simulink model "que5_2"  (R2023a)
settings: Solver=VariableStepAuto  StartTime=0.0  StopTime=150  RelTol=1e-3
values from neighbouring files (symbols this model uses):
  A = [0 1 0 0 ... (first row only)    [que5_1.m]    (also in que5_1_1.m; que5_4.m; que6_1.m = [0 1 0; que6_2_sim_input.m = [0 1 0;0 0 1;0 0 -0.5])
  B = [0 ... (first row only)    [que5_1.m]    (also in que5_1_1.m; que5_4.m; que6_1.m = [0 0 0.5]'; que6_2_sim_input.m = [0;0;0.5])
  C = [1,0, 0, 0 ... (first row only)    [que5_1.m]    (also in que5_1_1.m; que5_4.m = [1, 0, 0, 0]; que6_1.m = [1 0 0; que6_2_sim_input.m = [1 0 0)
  g = 9.8    [que5_1.m]    (also in que5_1_1.m; que5_4.m)
  I = 1/3*m*l^2    (= 0.00833333333333)    [que5_1.m]    (also in que5_1_1.m; que5_4.m)
  l = 0.5    [que5_1.m]    (also in que5_1_1.m; que5_4.m)
  m = 0.1    [que5_1.m]    (also in que5_1_1.m; que5_4.m)
  M = 2    [que5_1.m]    (also in que5_1_1.m; que5_4.m)
settings Model: Creator=Hasee  LastModifiedBy=Administrator

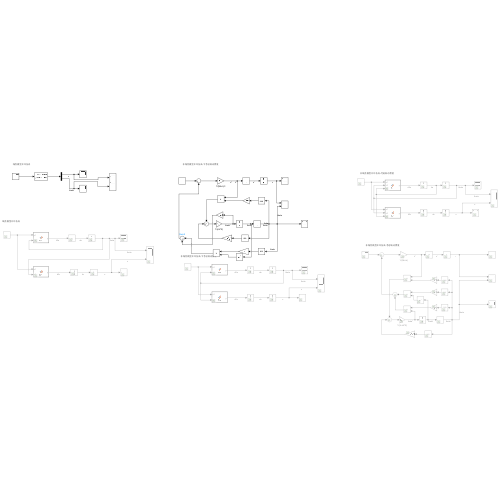
[thumbnail: Simulink's stored preview of the top-level diagram]
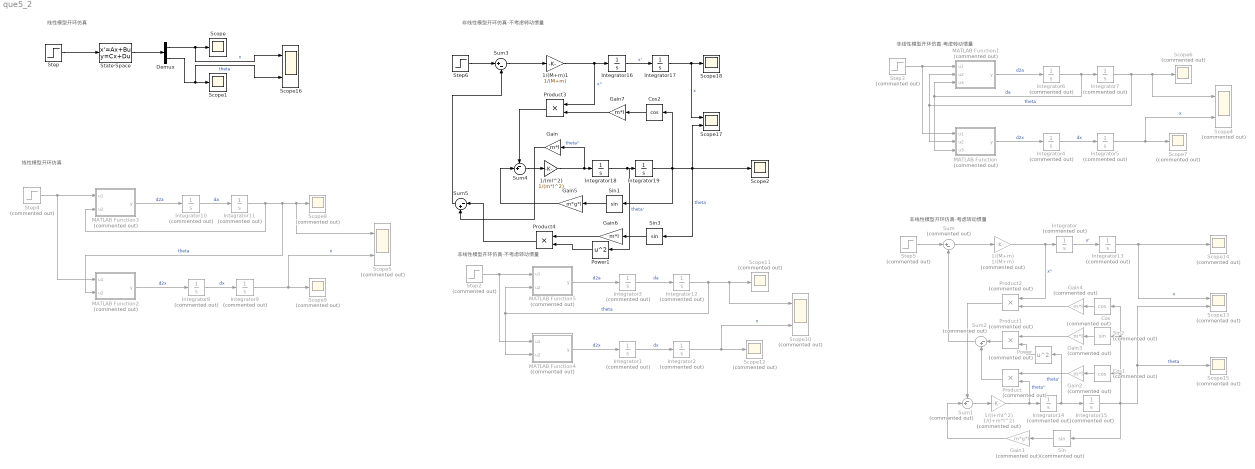
== system que5_2 ==
  note: 线性模型开环仿真
  note: 线性模型开环仿真
  note: 非线性模型开环仿真-不考虑转动惯量
  note: 非线性模型开环仿真-不考虑转动惯量
  note: 非线性模型开环仿真-考虑转动惯量
  note: 非线性模型开环仿真-考虑转动惯量
  1/(I+ml^2) : Gain  Commented=on  Gain=1/(I+m*l^2)
  1/(M+m) : Gain  Commented=on  Gain=1/(M+m)
  1/(M+m)1 : Gain  Gain=1/(M+m)
  1/(ml^2) : Gain  Gain=1/(m*l^2)
  Cos : Trigonometry  Commented=on  Operator=cos
  Cos1 : Trigonometry  Commented=on  Operator=cos
  Cos2 : Trigonometry  Operator=cos
  Demux : Demux  Outputs=2
  Gain : Gain  Gain=m*l
  Gain1 : Gain  Commented=on  Gain=m*g*l
  Gain2 : Gain  Commented=on  Gain=m*l
  Gain3 : Gain  Commented=on  Gain=m*l
  Gain4 : Gain  Commented=on  Gain=m*l
  Gain5 : Gain  Gain=m*g*l
  Gain6 : Gain  Gain=m*l
  Gain7 : Gain  Gain=m*l
  Integrator{,1..15} (16 alike) : Integrator  Commented=on
  Integrator{16..19} (4 alike) : Integrator
  MATLAB Function : MATLAB Function  Commented=on  TreatAsAtomicUnit=on
  MATLAB Function1 : MATLAB Function  Commented=on  TreatAsAtomicUnit=on
  MATLAB Function2 : MATLAB Function  Commented=on  TreatAsAtomicUnit=on
  MATLAB Function3 : MATLAB Function  Commented=on  TreatAsAtomicUnit=on
  MATLAB Function4 : MATLAB Function  Commented=on  TreatAsAtomicUnit=on
  MATLAB Function5 : MATLAB Function  Commented=on  TreatAsAtomicUnit=on
  Power : Math  Commented=on  Operator=square
  Power1 : Math  Operator=square
  Product : Product  Commented=on
  Product1 : Product  Commented=on
  Product2 : Product  Commented=on
  Product3 : Product
  Product4 : Product
  Scope{,1..2,18} (4 alike) : Scope
  Scope{4..5,10,13} (4 alike) : Scope  Commented=on  NumInputPorts=2
  Scope{6..9,11..12,14..15} (8 alike) : Scope  Commented=on
  Scope16 : Scope  NumInputPorts=2
  Scope17 : Scope  NumInputPorts=2
  Sin : Trigonometry  Commented=on
  Sin1 : Trigonometry
  Sin2 : Trigonometry  Commented=on
  Sin3 : Trigonometry
  State-Space : StateSpace  A=A  B=B  C=C  D=[0 0]'  InitialCondition=0
  Step : Step  Time=10  SampleTime=0
  Step{2..5} (4 alike) : Step  Commented=on  SampleTime=0
  Step6 : Step  SampleTime=0
  Sum : Sum  Commented=on  Inputs=|+-
  Sum1 : Sum  Commented=on  Inputs=-+|
  Sum2 : Sum  Commented=on  Inputs=|-+
  Sum3 : Sum  Inputs=|+-
  Sum4 : Sum  Inputs=-+|
  Sum5 : Sum  Inputs=|-+
  wires:
  Step/1 -> State-Space/1
  Demux/1 -> Scope16/1, Scope/1  "x"
  Demux/2 -> Scope16/2, Scope1/1  "theta"
  State-Space/1 -> Demux/1
  Integrator4/1 -> Integrator5/1  "dx"
  Integrator6/1 -> MATLAB Function/3(u3), MATLAB Function1/3(u3), Integrator7/1  "da"
  Integrator5/1 -> Scope4/2, Scope7/1  "x"
  Integrator7/1 -> MATLAB Function/2(u2), MATLAB Function1/2(u2), Scope4/1, Scope6/1  "theta"
  Step3/1 -> MATLAB Function/1(u1), MATLAB Function1/1(u1)
  MATLAB Function/1(y) -> Integrator4/1  "d2x"
  MATLAB Function1/1(y) -> Integrator6/1  "d2a"
  MATLAB Function3/1(y) -> Integrator10/1  "d2a"
  Integrator9/1 -> Scope5/2, Scope9/1  "x"
  Integrator8/1 -> Integrator9/1  "dx"
  Integrator10/1 -> Integrator11/1  "da"
  Step4/1 -> MATLAB Function2/1(u1), MATLAB Function3/1(u1)
  MATLAB Function2/1(y) -> Integrator8/1  "d2x"
  Integrator11/1 -> MATLAB Function3/2(u2), MATLAB Function2/2(u2), Scope5/1, Scope8/1  "theta"
  MATLAB Function5/1(y) -> Integrator3/1  "d2a"
  Integrator12/1 -> MATLAB Function4/2(u2), MATLAB Function5/2(u2), Scope10/1, Scope11/1  "theta"
  Integrator3/1 -> Integrator12/1  "da"
  Integrator2/1 -> Scope10/2, Scope12/1  "x"
  Step2/1 -> MATLAB Function4/1(u1), MATLAB Function5/1(u1)
  MATLAB Function4/1(y) -> Integrator1/1  "d2x"
  Integrator1/1 -> Integrator2/1  "dx"
  Integrator15/1 -> Scope15/1, Scope13/2, Cos/1, Sin2/1, Cos1/1, Sin/1  "theta"
  Product2/1 -> Sum1/1
  Sin/1 -> Gain1/1
  Product1/1 -> Sum2/1
  Cos1/1 -> Gain2/1
  Cos/1 -> Gain4/1
  Power/1 -> Product1/2
  Product/1 -> Sum2/2
  Integrator13/1 -> Scope14/1, Scope13/1  "x"
  Sin2/1 -> Gain3/1
  Integrator14/1 -> Integrator15/1, Power/1  "theta'"
  Gain4/1 -> Product2/2
  Gain2/1 -> Product/1
  1/(M+m)/1 -> Product2/1, Integrator/1  "x''"
  Gain3/1 -> Product1/1
  Step5/1 -> Sum/1
  Integrator/1 -> Integrator13/1  "x'"
  1/(I+ml^2)/1 -> Product/2, Integrator14/1  "theta''"
  Sum1/1 -> 1/(I+ml^2)/1
  Gain1/1 -> Sum1/2
  Sum/1 -> 1/(M+m)/1
  Sum2/1 -> Sum/2
  Step6/1 -> Sum3/1
  Sum3/1 -> 1/(M+m)1/1
  Sum4/1 -> 1/(ml^2)/1
  Integrator16/1 -> Integrator17/1  "x'"
  1/(ml^2)/1 -> Gain/1, Integrator18/1  "theta''"
  Integrator18/1 -> Power1/1, Integrator19/1  "theta'"
  Gain5/1 -> Sum4/2
  Integrator17/1 -> Scope18/1, Scope17/1  "x"
  Sin1/1 -> Gain5/1
  Gain/1 -> Sum5/2
  Gain7/1 -> Product3/2
  1/(M+m)1/1 -> Product3/1, Integrator16/1  "x''"
  Product3/1 -> Sum4/1
  Cos2/1 -> Gain7/1
  Integrator19/1 -> Scope17/2, Scope2/1, Sin3/1, Cos2/1, Sin1/1  "theta"
  Sin3/1 -> Gain6/1
  Gain6/1 -> Product4/1
  Power1/1 -> Product4/2
  Product4/1 -> Sum5/1
  Sum5/1 -> Sum3/2

== matlab function que5_2/MATLAB Function ==
  data: u1 input; u2 input; y output; u3 input
function y = fcn(u1,u2,u3)
    %y = (u1-0.98*sin(u2)) / (2.1-0.1*cos(u2));
    y = (0.1*9.8*sin(u2)*cos(u2)-0.05*u3*u3*sin(u2))/(2+0.1*sin(u2)*sin(u2))+(1/(2+0.1*sin(u2)*sin(u2))*u1)
end

== matlab function que5_2/MATLAB Function2 ==
  data: u1 input; u2 input; y output
function y = fcn(u1,u2)
    y = (u1-0.98*u2)/2;
end

== matlab function que5_2/MATLAB Function3 ==
  data: u1 input; u2 input; y output
function y = fcn(u1,u2)
    y = 2.1*9.8*u2-u1;
end

== matlab function que5_2/MATLAB Function4 ==
  data: u1 input; u2 input; y output
function y = fcn(u1,u2)
    %y = (u1-0.98*sin(u2)) / (2.1-0.1*cos(u2));
    y = (u1-0.98*sin(u2))/(2.1-0.1*cos(u2))
end

== matlab function que5_2/MATLAB Function5 ==
  data: u1 input; u2 input; y output
function y = fcn(u1,u2)
    %y = (u1 - (u1-0.98*sin(u2))/(2.1-0.1*cos(u2)))/0.05;
    y = (u1-((u1-0.98*sin(u2))/(2.1-0.1*cos(u2))))/0.05
end

== matlab function que5_2/MATLAB Function1 ==
  data: u1 input; u2 input; y output; u3 input
function y = fcn(u1,u2,u3)
    %y = (u1 - (u1-0.98*sin(u2))/(2.1-0.1*cos(u2)))/0.05;
    y = (2.1*9.8*sin(u2)-0.05*u3*u3*sin(u2)*cos(u2))/(1+0.05*sin(u2)*sin(u2))+(cos(u2)/(1+0.05*sin(u2)*sin(u2))*u1);
end
